simulink model "Main1"  (R2017b)
settings: Solver=ode15s  StartTime=0.0  StopTime=t_end  FixedStep=.0001  MaxStep=st  RelTol=1e-3  EnableMultiTasking=on
values from neighbouring files (symbols this model uses):
  A = eye(16,16)    [full_input_list.m]
  B = zeros(16,1)    [full_input_list.m]
  C = blkdiag(eye(3,3),zeros(3,3),eye(10,10))    [full_input_list.m]
  deltaT = 0.00001    (= 1e-05)    [full_input_list.m]
  H = C    [full_input_list.m]
  I_UD = [0.032808359, 0.000617048, 0.000049185;      0.000617048, 0.032531573, 0.000060042;      0.000049185, 0.000060042, 0.007799591]    [full_input_list.m]
  kd = 0.5    [full_input_list.m]    (also in initACS.m = 0.01)
  kd_UD_detumble = 6e-3    (= 0.006)    [full_input_list.m]
  kd_UD_slew = epsilon_UD_slew*.3    (= 0.003)    [full_input_list.m]
  kd_UD_spinUp = epsilon_UD_spinUp*0.025    (= 0.00025)    [full_input_list.m]
  kp = 1    [full_input_list.m]    (also in initACS.m = 0.01)
  kp_UD_slew = epsilon_UD_slew^2*.01    (= 1e-06)    [full_input_list.m]
  kp_UD_spinUp = epsilon_UD_spinUp^2*.05    (= 5e-06)    [full_input_list.m]
  magMomentMax_B = sat2CoilArea.*sat2n.*currentMax_B    [full_input_list.m]
  omega_cmd_N = 1e-1*[1 1 -.6]'    [full_input_list.m]
  omega_spinUp_MAG = 0.05    [full_input_list.m]
  OpModes = [0 0 0]    [full_input_list.m]
  OpTimes = [0 1 2]    [full_input_list.m]
  q4_cmd_init = [q4_cmd_init(2:4); q4_cmd_init(1)]    [full_input_list.m]
  Q_k = zeros(16,16)    [full_input_list.m]
  R = R_k    [full_input_list.m]
  sat2CoilArea = 0.8*[0.02; 0.02; 0.01]    [full_input_list.m]
  sat2n = [0; 100; 100]    [full_input_list.m]
  sat2Resistance = sat2WireLength.*sat2WireResistivity./sat2WireArea    [full_input_list.m]
  SeperationTime = 30000    [full_input_list.m]
  spinAxis_B = [1 0 0]    [full_input_list.m]
  st = 1/freq    (= 0.0125)    [full_input_list.m]    (also in initSimulink.m)
  u_k = zeros(16,1)    [full_input_list.m]
  w_k = zeros(16,1)    [full_input_list.m]
  Z_k = zeros(16,1)    [full_input_list.m]
undefined symbols (not defined in the file or in its folder): DiscIntNeverNeededParam, G_igrf, gyro_DCM_BS, H_igrf, I_B, IAU, Kschmidt, mag_variance, R_mean
libraries: aerolibutil x36, vrlib x31, SimMainLibrary x27, simulink x22, dspmathops x6, sharedtransform x4, sharedutil x2, dspinverses x2, dspmtrx3 x1, aerolibtransform2 x1, aerolibgravity2 x1, lib_violet_env x1
(part 1 of 3)
settings Model: Creator=dtk42  LastModifiedBy=vtroo
settings SolverCC: ZeroCrossAlgorithm=Adaptive
settings OptimizationCC: LifeSpan=inf
settings DebuggingCC: SFUnexpectedBacktrackingDiag=warning  SFNoUnconditionalDefaultTransitionDiag=warning  SFExecutionAtInitializationDiag=none
settings CodeAppCC: StateflowObjectComments=on
settings GRTTargetCC: TargetLangStandard=C89/C90 (ANSI)
settings ConfigComp: CovMetricSettings=dw  CovHtmlReporting=on  CovSaveCumulativeToWorkspaceVar=on  CovSaveSingleToWorkspaceVar=on  CovExternalEMLEnable=off
settings SimscapeCC: SimscapeNormalizeSystem=off
settings ExplorerConfigSet: InternalSimMechanicsExplorerSettings="<ExplorerConfiguration><canonicalview>default</canonicalview><AnimationSetting><BasePlaybackSpeed>1.0</BasePlaybackSpeed><PlaybackSpeedFactor>0.125</PlaybackSpeedFactor></AnimationSetting><TilePanel><TileInfo><Tiles Columns=\"1\" Count=\"1\" Rows=\"1\"><Column Weight=\"1\"/><Row Weight=\"1\"/><Tile Height=\"1\" Width=\"1\" X=\"0\" Y=\"0\"/></Tiles></TileInfo><SceneInfo><SceneViewer><BGColor><R>0.60000002384185791</R><G>0.60000002384185791</G><B>0.60000002384185791</B></BGColor><Camera><DoPerspective>on</DoPerspective><Position><X>0.299996941150711738</X><Y>-0.0249603631658691372</Y><Z>0.248754528744442288</Z></Position><Center><X>-0.199992462724818743</X><Y>0.0615041817400976409</Y><Z>-0.612949874450989807</Z></Center><Up><X>0.866031521373320734</X><Y>0.049918851895640326</Y><Z>-0.49749121822724951</Z></Up><ViewLimDist>1</ViewLimDist><YLim>0.466307658154998583</YLim><XLim>1.03172600323492714</XLim></Camera></SceneViewer></SceneInfo></TilePanel><MechEditorPanel><Cameras><Camera><Id>Camera1</Id><Value><Name>Camera1</Name><NativeCamera><PositionTrackingFeature>Dynamics_Configurable_System1.Three_Link_Simscape_Model.Camera1_Frame.F</PositionTrackingFeature><CenterTrackingFeature>Dynamics_Configurable_System1.Three_Link_Simscape_Model.Camera1_Frame.F</CenterTrackingFeature><UpVectorTrackingFeature>Dynamics_Configurable_System1.Three_Link_Simscape_Model.Camera1_Frame.F</UpVectorTrackingFeature><CenterTrackingOrigin>off</CenterTrackingOrigin><CenterTrackingDirection>-Z</CenterTrackingDirection><UpVectorTrackingDirection>+X</UpVectorTrackingDirection></NativeCamera></Value></Camera></Cameras><GfxPanelCameraMap><MapElement CameraMLId=\"Camera1\" GfxPanelIndex=\"0\"/></GfxPanelCameraMap><VideoCreator><PlaybackSpeedRatio>0.25</PlaybackSpeedRatio><FrameRate>30</FrameRate><VideoFormat>Motion JPEG AVI</VideoFormat><FrameSize>[800 600]</FrameSize></VideoCreator></MechEditorPanel></ExplorerConfiguration>"

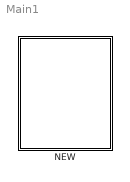
== system Main1 ==
  NEW : Subsystem

== system Main1/NEW ==
  note: CUGravity Top Level Simulation
  note: Feeding exact telemetry from dynamics into FC. Substitute this for EKF output until estimation is ready for implementation.
  Dynamics Configurable System2 : Subsystem  BlockChoice=Three Link Simscape Model
      link override Extendable Single  Link Simscape /s_teth_init2: PxPositionTargetSpecify=on  PxPositionTargetValue=eps
      link override Single Link Simscape Model/s_teth_init: PxPositionTargetSpecify=on  PxPositionTargetValue=eps  PyPositionTargetSpecify=on  PyPositionTargetValue=eps  PzPositionTargetSpecify=on  PzPositionTargetValue=eps
      link override Single Link Simscape Model/s_teth_init2: PxPositionTargetSpecify=on  PxPositionTargetValue=eps  PyPositionTargetSpecify=on  PyPositionTargetValue=eps  PzPositionTargetSpecify=on  PzPositionTargetValue=eps
      link override Three Link Simscape Model/Kane Damper 1: SerializedFrames=<Frames><Frame><Id>Frame1</Id><Value><Name>F1</Name><Origin><Source>GeometricFeature</Source><FeatureName>+z surface</FeatureName></Origin><PrimaryAxis><DefinedDirection>+Z</DefinedDirection><Source>ReferenceFrame</Source><SourceDirection>+Z</SourceDirection><FeatureName></FeatureName></PrimaryAxis><SecondaryAxis><DefinedDirection>+X</DefinedDirection><Source>ReferenceFrame</Source><SourceDirection>+X</SourceDirection><FeatureName></FeatureName></SecondaryAxis></Value></Frame></Frames>
      link override Three Link Simscape Model/Kane Damper 2: SerializedFrames=<Frames><Frame><Id>Frame1</Id><Value><Name>F1</Name><Origin><Source>GeometricFeature</Source><FeatureName>-z surface</FeatureName></Origin><PrimaryAxis><DefinedDirection>+Z</DefinedDirection><Source>ReferenceFrame</Source><SourceDirection>+Z</SourceDirection><FeatureName></FeatureName></PrimaryAxis><SecondaryAxis><DefinedDirection>+X</DefinedDirection><Source>ReferenceFrame</Source><SourceDirection>+X</SourceDirection><FeatureName></FeatureName></SecondaryAxis></Value></Frame></Frames>  GeometryShape=Brick  BrickDimensions=[kane_radius kane_radius kane_height]
      link override Undeployed Model/Center Sat1: GraphicDiffuseColor=[0.0 0.8 0.8]  GraphicOpacity=.5  SerializedFrames=<Frames><Frame><Id>Frame1</Id><Value><Name>PosZ</Name><Origin><Source>GeometricFeature</Source><FeatureName>+z surface</FeatureName></Origin><PrimaryAxis><DefinedDirection>+Z</DefinedDirection><Source>ReferenceFrame</Source><SourceDirection>+Z</SourceDirection><FeatureName></FeatureName></PrimaryAxis><SecondaryAxis><DefinedDirection>+X</DefinedDirection><Source>ReferenceFrame</Source><SourceDirection>+X</SourceDirection><FeatureName></FeatureName></SecondaryAxis></Value></Frame><Frame><Id>Frame2</Id><Value><Name>NegZ</Name><Origin><Source>GeometricFeature</Source><FeatureName>-z surface</FeatureName></Origin><PrimaryAxis><DefinedDirection>+Z</DefinedDirection><Source>ReferenceFrame</Source><SourceDirection>+Z</SourceDirection><FeatureName></FeatureName></PrimaryAxis><SecondaryAxis><DefinedDirection>+X</DefinedDirection><Source>ReferenceFrame</Source><SourceDirection>+X</SourceDirection><FeatureName></FeatureName></SecondaryAxis></Value></Frame><Frame><Id>Frame7</Id><Value><Name>PosX</Name><Origin><Source>GeometricFeature</Source><FeatureName>+x surface</FeatureName></Origin><PrimaryAxis><DefinedDirection>+Z</DefinedDirection><Source>ReferenceFrame</Source><SourceDirection>+Z</SourceDirection><FeatureName></FeatureName></PrimaryAxis><SecondaryAxis><DefinedDirection>+X</DefinedDirection><Source>ReferenceFrame</Source><SourceDirection>+X</SourceDirection><FeatureName></FeatureName></SecondaryAxis></Value></Frame><Frame><Id>Frame8</Id><Value><Name>COM</Name><Origin><Source>CenterOfMassFrame</Source><FeatureName></FeatureName></Origin><PrimaryAxis><DefinedDirection>+Z</DefinedDirection><Source>ReferenceFrame</Source><SourceDirection>+Z</SourceDirection><FeatureName></FeatureName></PrimaryAxis><SecondaryAxis><DefinedDirection>+X</DefinedDirection><Source>ReferenceFrame</Source><SourceDirection>+X</SourceDirection><FeatureName></FeatureName></SecondaryAxis></Value></Frame></Frames>
      link override Undeployed Model/EndSat3: GraphicOpacity=.5  GraphicDiffuseColor=[1.0 0.0 0.0]
      link override Undeployed Model/EndSat4: GraphicOpacity=.5  GraphicDiffuseColor=[1.0 0.0 0.0]
      settings: AttributesFormatString=%<BlockChoice>  TemplateBlock=SimMainLibrary/Dynamics Configurable System  MemberBlocks="Extendable Single  Link Simscape ,Single Link Simscape Model,Three Link Simscape Model,Undeployed Model"
  Flight Computers1 : Subsystem
  Memory2 : Memory  InheritSampleTime=on
  Memory3 : Memory  InheritSampleTime=on
  Rate Transition3 : RateTransition  OutPortSampleTime=st
  Rate Transition4 : RateTransition  OutPortSampleTime=st
  Scope : Scope
  Scopes1 : Subsystem
  Sensors1 : Subsystem  mask(State Estimation){}
      mask help: This block uses the plant model calculated state (input) and adds sensor noise to the system to calculate the estimated state (output). The middle satellite has a more extensive set of calculations required to complete the state estimation, than do the end satellites. All three satellites compute the accelerometer, magnetometer, angular velocity, and sun sensor vector measurements. The middle satellite performs additional calculations to accurately measure simulation time and inertial position of the center of mass.
  To Workspace3 : ToWorkspace  VariableName=stateArr1  SaveFormat=Timeseries  SampleTime=-1
  To Workspace5 : ToWorkspace  VariableName=stateEstimation1  SaveFormat=Timeseries  SampleTime=-1
  wires:
  Dynamics Configurable System2/1(State k+1) -> To Workspace3/1, Memory2/1, Scopes1/2(state)
  Flight Computers1/2(PwbMEX) -> Memory3/1
  Dynamics Configurable System2/2(DEBUG) -> Scope/1
  Rate Transition4/1 -> Flight Computers1/2(TEMP_State)
  Flight Computers1/3(StateEst) -> To Workspace5/1
  Rate Transition3/1 -> Flight Computers1/1(Sensor Data)
  Sensors1/1(Observation) -> Rate Transition3/1
  Memory2/1 -> Sensors1/1(State), Rate Transition4/1
  Flight Computers1/1(FC Outputs) -> Dynamics Configurable System2/1(Actuation Cmds), Scopes1/1(torque_N)
  Memory3/1 -> Flight Computers1/3(PwbMEXin)

== system Main1/NEW/Dynamics Configurable System2 ==
  Actuation Cmds : Inport
  Three Link Simscape Model : SimMainLibrary/Three Link Simscape Model
      settings: SourceProductName=CUGravity Library
  State k+1 : Outport
  DEBUG : Outport  Port=2
  wires:
  Actuation Cmds/1 -> Three Link Simscape Model/1
  Three Link Simscape Model/1 -> State k+1/1
  Three Link Simscape Model/2 -> DEBUG/1

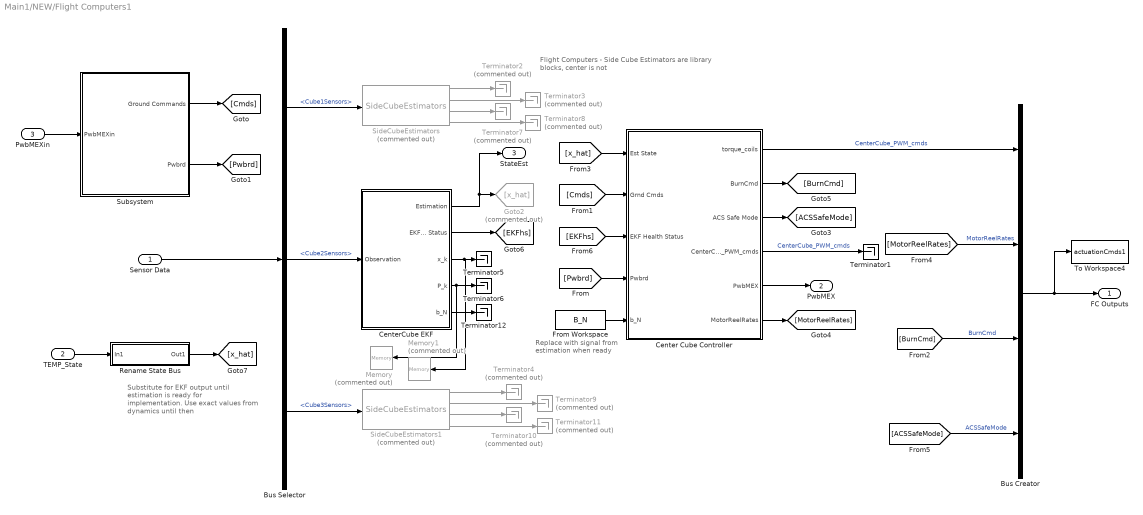
== system Main1/NEW/Flight Computers1 ==
  note: Substitute for EKF output until estimation is ready for implementation. Use exact values from dynamics until then
  note: Flight Computers
      | - Side Cube Estimators are library blocks, center is not
  note: Replace with signal from estimation when ready
  Sensor Data : Inport
  TEMP_State : Inport  Port=2
  PwbMEXin : Inport  Port=3
  Bus Creator : BusCreator  Inputs=4
  Bus Selector : BusSelector  OutputSignals=Cube1Sensors,Cube2Sensors,Cube3Sensors
  Center Cube Controller : Subsystem
  CenterCube EKF : Subsystem
  From Workspace : FromWorkspace  VariableName=B_N  SampleTime=0
  Goto2 : Goto  Commented=on  GotoTag=x_hat
  Memory : Memory  Commented=on
  Memory1 : Memory  Commented=on
  Rename State Bus : Subsystem
  SideCubeEstimators : SimMainLibrary/SideCubeEstimators  Commented=on
      settings: SourceProductName=CUGravity Library
  SideCubeEstimators1 : SimMainLibrary/SideCubeEstimators  Commented=on
      settings: SourceProductName=CUGravity Library
  Subsystem : Subsystem
  Terminator{1,5..6,12} (4 alike) : Terminator
  Terminator{2..4,7..11} (8 alike) : Terminator  Commented=on
  To Workspace4 : ToWorkspace  VariableName=actuationCmds1  SaveFormat=Timeseries  SampleTime=-1
  FC Outputs : Outport
  PwbMEX : Outport  Port=2
  StateEst : Outport  Port=3
  wires:
  Sensor Data/1 -> Bus Selector/1
  Bus Selector/1 -> SideCubeEstimators/1  "<Cube1Sensors>"
  Bus Selector/2 -> CenterCube EKF/1(Observation)  "<Cube2Sensors>"
  Bus Selector/3 -> SideCubeEstimators1/1  "<Cube3Sensors>"
  SideCubeEstimators/1 -> Terminator2/1
  Bus Creator/1 -> To Workspace4/1, FC Outputs/1
  Subsystem/1(Ground Commands) -> [Cmds]
  [Cmds] -> Center Cube Controller/2(Grnd Cmds)
  Center Cube Controller/3(ACS Safe Mode) -> [ACSSafeMode]
  Center Cube Controller/2(BurnCmd) -> [BurnCmd]
  [BurnCmd] -> Bus Creator/3  "BurnCmd"
  CenterCube EKF/2(EKF Health Status) -> [EKFhs]
  [EKFhs] -> Center Cube Controller/3("EKF Health Status ")
  Subsystem/2(Pwbrd) -> [Pwbrd]
  [Pwbrd] -> Center Cube Controller/4(Pwbrd)
  Center Cube Controller/5(PwbMEX) -> PwbMEX/1
  CenterCube EKF/1(Estimation) -> Goto2/1, StateEst/1
  [x_hat] -> Center Cube Controller/1(Est State)
  Center Cube Controller/4(CenterCube_PWM_cmds) -> Terminator1/1  "CenterCube_PWM_cmds"
  SideCubeEstimators/2 -> Terminator3/1
  CenterCube EKF/3(x_k) -> Memory1/1, Terminator5/1
  CenterCube EKF/4(P_k) -> Terminator6/1, Memory/1
  SideCubeEstimators/3 -> Terminator7/1
  SideCubeEstimators/4 -> Terminator8/1
  SideCubeEstimators1/1 -> Terminator4/1
  SideCubeEstimators1/2 -> Terminator9/1
  SideCubeEstimators1/3 -> Terminator10/1
  SideCubeEstimators1/4 -> Terminator11/1
  [ACSSafeMode] -> Bus Creator/4  "ACSSafeMode"
  Center Cube Controller/6(MotorReelRates) -> [MotorReelRates]
  [MotorReelRates] -> Bus Creator/2  "MotorReelRates"
  Center Cube Controller/1(torque_coils) -> Bus Creator/1  "CenterCube_PWM_cmds"
  From Workspace/1 -> Center Cube Controller/5(b_N)
  CenterCube EKF/5(b_N) -> Terminator12/1
  TEMP_State/1 -> Rename State Bus/1(In1)
  Rename State Bus/1(Out1) -> [x_hat]
  PwbMEXin/1 -> Subsystem/1(PwbMEXin)

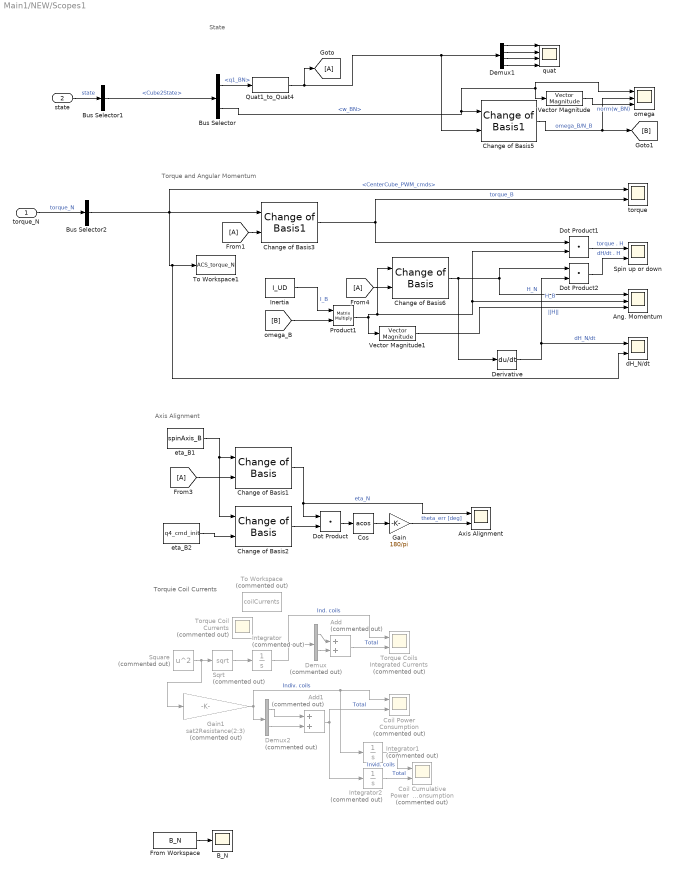
== system Main1/NEW/Scopes1 ==
  note: State
  note: Torque and Angular Momentum
  note: Axis Alignment
  note: Torquie Coil Currents
  torque_N : Inport
  state : Inport  Port=2
  Add : Sum  Commented=on
  Add1 : Sum  Commented=on
  Ang. Momentum : Scope  NumInputPorts=3
  Axis Alignment : Scope  NumInputPorts=2
  B_N : Scope
  Bus Selector : BusSelector  OutputSignals=q1_BN,w_BN
  Bus Selector1 : BusSelector  OutputSignals=Cube2State
  Bus Selector2 : BusSelector  OutputSignals=CenterCube_PWM_cmds
  Change of Basis1 : SimMainLibrary/Change of Basis
      settings: SourceProductName=CUGravity Library
  Change of Basis2 : SimMainLibrary/Change of Basis
      settings: SourceProductName=CUGravity Library
  Change of Basis3 : SimMainLibrary/Change of Basis1
      settings: SourceProductName=CUGravity Library
  Change of Basis5 : SimMainLibrary/Change of Basis1
      settings: SourceProductName=CUGravity Library
  Change of Basis6 : SimMainLibrary/Change of Basis
      settings: SourceProductName=CUGravity Library
  Coil Cumulative Power  Consumption : Scope  Commented=on  NumInputPorts=2
  Coil Power Consumption : Scope  Commented=on  NumInputPorts=2
  Cos : Trigonometry  Operator=acos
  Demux : Demux  Commented=on  Outputs=2
  Demux1 : Demux
  Demux2 : Demux  Commented=on  Outputs=2
  Derivative : Derivative
  Dot Product : DotProduct  InputSameDT=on  OutDataTypeStr=Inherit: Inherit via internal rule
  Dot Product1 : DotProduct  InputSameDT=on  OutDataTypeStr=Inherit: Inherit via internal rule
  Dot Product2 : DotProduct  InputSameDT=on  OutDataTypeStr=Inherit: Inherit via internal rule
  From Workspace : FromWorkspace  VariableName=B_N  SampleTime=0
  Gain : Gain  Gain=180/pi
  Gain1 : Gain  Commented=on  Gain=sat2Resistance(2:3)
  Inertia : Constant  Value=I_UD
  Integrator : Integrator  Commented=on
  Integrator1 : Integrator  Commented=on
  Integrator2 : Integrator  Commented=on
  Product1 : Product  Multiplication=Matrix(*)
  Quat1_to_Quat4 : SimMainLibrary/Quat1_to_Quat4
      settings: SourceProductName=CUGravity Library
  Spin up or down : Scope  NumInputPorts=2
  Sqrt : Sqrt  Commented=on  SaturateOnIntegerOverflow=on
  Square : Math  Commented=on  Operator=square  RndMeth=Zero  SaturateOnIntegerOverflow=on
  To Workspace : ToWorkspace  Commented=on  VariableName=coilCurrents  SaveFormat=Timeseries  SampleTime=-1
  To Workspace1 : ToWorkspace  VariableName=ACS_torque_N  SaveFormat=Timeseries  SampleTime=-1
  Torque Coil Currents : Scope  Commented=on
  Torque Coils Integrated Currents : Scope  Commented=on  NumInputPorts=2
  Vector Magnitude : SimMainLibrary/Vector Magnitude
      settings: SourceProductName=CUGravity Library
  Vector Magnitude1 : SimMainLibrary/Vector Magnitude
      settings: SourceProductName=CUGravity Library
  dH_N/dt : Scope  NumInputPorts=2
  eta_B1 : Constant  Value=spinAxis_B
  eta_B2 : Constant  Value=q4_cmd_init
  omega : Scope  NumInputPorts=3
  quat : Scope  NumInputPorts=4
  torque : Scope  NumInputPorts=2
  wires:
  ? -> To Workspace/1, Square/1, Torque Coil Currents/1
  Integrator/1 -> Demux/1, Torque Coils Integrated Currents/1  "Ind. coils"
  Cos/1 -> Gain/1
  Change of Basis1/1 -> Dot Product/1, Axis Alignment/1  "eta_N"
  eta_B1/1 -> Change of Basis2/1, Change of Basis1/1
  Change of Basis2/1 -> Dot Product/2
  eta_B2/1 -> Change of Basis2/2
  [A] -> Change of Basis1/2
  Dot Product/1 -> Cos/1
  Gain/1 -> Axis Alignment/2  "theta_err [deg]"
  Bus Selector2/1 -> dH_N/dt/2, To Workspace1/1, torque/1, Change of Basis3/1  "<CenterCube_PWM_cmds>"
  [B] -> Product1/2
  Dot Product1/1 -> Spin up or down/1  "torque . H"
  Derivative/1 -> dH_N/dt/1, Dot Product2/2  "dH_N/dt"
  Vector Magnitude1/1 -> Ang. Momentum/3  "||H||"
  [A] -> Change of Basis3/2
  Product1/1 -> Change of Basis6/1, Ang. Momentum/2, Dot Product1/2, Vector Magnitude1/1  "H_B"
  Inertia/1 -> Product1/1  "I_B"
  Change of Basis3/1 -> Dot Product1/1, torque/2  "torque_B"
  [A] -> Change of Basis6/2
  Change of Basis6/1 -> Derivative/1, Dot Product2/1, Ang. Momentum/1  "H_N"
  Demux1/2 -> quat/2
  Demux1/3 -> quat/3
  Demux1/4 -> quat/4
  Bus Selector/2 -> Change of Basis5/1, Vector Magnitude/1, omega/1  "<w_BN>"
  Change of Basis5/1 -> omega/2, [B]  "omega_B/N_B"
  Bus Selector/1 -> Quat1_to_Quat4/1  "<q1_BN>"
  Vector Magnitude/1 -> omega/3  "norm(w_BN)"
  Demux1/1 -> quat/1
  Square/1 -> Gain1/1, Sqrt/1
  Sqrt/1 -> Integrator/1
  Demux/1 -> Add/1
  Demux/2 -> Add/2
  Add/1 -> Torque Coils Integrated Currents/2  "Total"
  Gain1/1 -> Integrator1/1, Coil Power Consumption/1, Demux2/1  "Indiv. coils"
  Demux2/1 -> Add1/1
  Demux2/2 -> Add1/2
  Add1/1 -> Integrator2/1, Coil Power Consumption/2  "Total"
  Integrator1/1 -> Coil Cumulative Power  Consumption/1  "Invid. coils"
  Integrator2/1 -> Coil Cumulative Power  Consumption/2  "Total"
  state/1 -> Bus Selector1/1  "state"
  Bus Selector1/1 -> Bus Selector/1  "<Cube2State>"
  Quat1_to_Quat4/1 -> [A], Change of Basis5/2, Demux1/1
  torque_N/1 -> Bus Selector2/1  "torque_N"
  Dot Product2/1 -> Spin up or down/2  "dH/dt . H"
  From Workspace/1 -> B_N/1

== system Main1/NEW/Sensors1 ==
  State : Inport
  Bus Creator1 : BusCreator  Inputs=3
  Bus Selector1 : BusSelector  OutputSignals=Cube1State,Cube2State,Cube3State
  Center Cube Sensors : Subsystem
  EndSat Sensor1 : Subsystem
  EndSat Sensor2 : Subsystem
  Observation : Outport
  wires:
  Bus Creator1/1 -> Observation/1
  Bus Selector1/1 -> EndSat Sensor2/1(State)  "<Cube1State>"
  EndSat Sensor2/1(Sensors) -> Bus Creator1/1  "Cube1Sensors"
  EndSat Sensor1/1(Sensors) -> Bus Creator1/3  "Cube3Sensors"
  Center Cube Sensors/1(Sensors) -> Bus Creator1/2  "Cube2Sensors"
  Bus Selector1/2 -> Center Cube Sensors/1(State)  "<Cube2State>"
  Bus Selector1/3 -> EndSat Sensor1/1(State)  "<Cube3State>"
  State/1 -> Bus Selector1/1

== system Main1/NEW/Flight Computers1/Center Cube Controller ==
  note: Why does torque coils suddenly become PWM?
  Est State : Inport
  Grnd Cmds : Inport  Port=2
  "EKF Health Status " : Inport  Port=3
  Pwbrd : Inport  Port=4
  b_N : Inport  Port=5
  Attitude Compensator : Subsystem
  Bus Selector : BusSelector  OutputSignals=w_BN_est
  Memory : Memory  InheritSampleTime=on
  Motor Control Placeholder : Subsystem  Commented=on
  Motor Controller Scope : Scope
  SafeMode : Subsystem
  "Sequential Motor Controller " : SimMainLibrary/Sequential Motor Controller
      settings: SourceProductName=CUGravity Library
  Terminator1 : Terminator
  Terminator2 : Terminator
  Terminator3 : Terminator
  Torque Coil Management : Subsystem
  torque_coils : Outport
  BurnCmd : Outport  Port=2
  ACS Safe Mode : Outport  Port=3
  CenterCube_PWM_cmds : Outport  Port=4
  PwbMEX : Outport  Port=5
  MotorReelRates : Outport  Port=6
  wires:
  Memory/1 -> SafeMode/3(Safe Mode In)
  Attitude Compensator/2(SepBurn) -> BurnCmd/1
  SafeMode/2(SafedSeperationBurn) -> Attitude Compensator/2(SafedSepBurn)
  SafeMode/3(SafedPos) -> Terminator3/1
  SafeMode/4(SafedVel) -> Terminator2/1
  Est State/1 -> SafeMode/2(EstState)
  SafeMode/1(SafedOpMode) -> "Sequential Motor Controller "/2, Motor Control Placeholder/2(SafedOpMode), Attitude Compensator/1(SafedOpMode)
  Grnd Cmds/1 -> SafeMode/1(GrndCmds)
  "EKF Health Status "/1 -> SafeMode/5("EKFhs ")
  Pwbrd/1 -> SafeMode/4(Pwbrd)
  Torque Coil Management/2(torque_coils) -> torque_coils/1
  Torque Coil Management/1(CenterCube_PWM_cmds) -> CenterCube_PWM_cmds/1
  Attitude Compensator/3(torque_N) -> Torque Coil Management/2(torque_N)
  SafeMode/5(Safed Att. State) -> Bus Selector/1, Torque Coil Management/1(Att. State), Attitude Compensator/3(Att. State)
  SafeMode/6(Safe Mode Out) -> Memory/1, ACS Safe Mode/1
  SafeMode/7(PwbMEX) -> PwbMEX/1
  Attitude Compensator/1(OpMode) -> Terminator1/1
  "Sequential Motor Controller "/1 -> MotorReelRates/1
  "Sequential Motor Controller "/2 -> Motor Controller Scope/1
  b_N/1 -> [B_N]
  [B_N] -> Attitude Compensator/4(B_N)
  [B_N] -> Torque Coil Management/3(B_N)
  Bus Selector/1 -> "Sequential Motor Controller "/1  "<w_BN_est>"

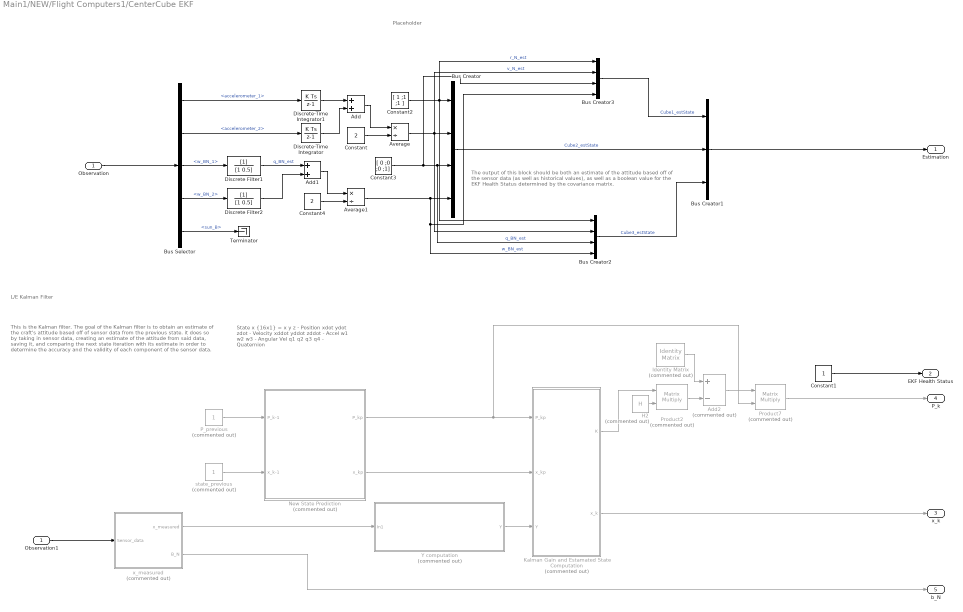
== system Main1/NEW/Flight Computers1/CenterCube EKF ==
  note: The output of this block should be both an estimate of the attitude based off of the sensor data (as well as historical values), as well as a boolean value for the EKF Health Status determined by the covariance matrix.
  note: Placeholder
  note: This is the Kalman filter. The goal of the Kalman filter is to obtain an estimate of the craft's attitude based off of sensor data from the previous state. it does so by taking in sensor data, creating an estimate of the attitude from said data, saving it, and comparing the next state iteration with its estimate in order to determine the accuracy and the validity of each component of the sensor data.
  note: L/E Kalman Filter
  note: State x {16x1} =
      | x y z - Position
      | xdot ydot zdot - Velocity
      | xddot yddot zddot - Accel
      | w1 w2 w3 - Angular Vel
      | q1 q2 q3 q4 - Quaternion
  Observation : Inport
  Add : Sum
  Add1 : Sum
  Add2 : Sum  Commented=on  Inputs=+-
  Average : Product  Inputs=*/
  Average1 : Product  Inputs=*/
  Bus Creator : BusCreator  Inputs=4
  Bus Creator1 : BusCreator  Inputs=3
  Bus Creator2 : BusCreator  Inputs=4
  Bus Creator3 : BusCreator  Inputs=4
  Bus Selector : BusSelector  OutputSignals=accelerometer_1,accelerometer_2,w_BN_1,w_BN_2,sun_B
  Constant : Constant  Value=2
  Constant1 : Constant
  Constant2 : Constant  Value=[ 1 ;1 ;1 ]
  Constant3 : Constant  Value=[ 0 ;0 ;0 ;1]
  Constant4 : Constant  Value=2
  Discrete Filter1 : DiscreteFilter
  Discrete Filter2 : DiscreteFilter
  Discrete-Time Integrator : DiscreteIntegrator  InitialConditionSetting=State (most efficient)  SampleTime=-1  ICPrevOutput=DiscIntNeverNeededParam  ICPrevScaledInput=DiscIntNeverNeededParam
  Discrete-Time Integrator1 : DiscreteIntegrator  InitialConditionSetting=State (most efficient)  SampleTime=-1  ICPrevOutput=DiscIntNeverNeededParam  ICPrevScaledInput=DiscIntNeverNeededParam
  H2 : Constant  Commented=on  Value=H
  Identity Matrix : dspmtrx3/Identity Matrix  Commented=on  Inherit=off  N=16  Ts=1  dataType=double  isSigned=on  wordLen=16  udDataType=sfix(16)  fracBitsMode=Best precision  numFracBits=15  OutDataTypeStr=double  LastOutDataTypeStr=double
      settings: SourceProductName=DSP System Toolbox
  Kalman Gain and Estamated State Computation : Subsystem  Commented=on
  "New State Prediction " : Subsystem  Commented=on
  Observation1 : InportShadow
  P_previous : Constant  Commented=on
  Product2 : Product  Commented=on  Multiplication=Matrix(*)
  Product7 : Product  Commented=on  Multiplication=Matrix(*)
  Terminator : Terminator
  Y computation : Subsystem  Commented=on
  state_previous : Constant  Commented=on
  x_measured : Subsystem  Commented=on
  Estimation : Outport
  EKF Health Status : Outport  Port=2
  x_k : Outport  Port=3
  P_k : Outport  Port=4
  b_N : Outport  Port=5
  wires:
  Bus Selector/2 -> Discrete-Time Integrator/1  "<accelerometer_2>"
  Discrete-Time Integrator/1 -> Add/2
  Bus Selector/4 -> Discrete Filter2/1  "<w_BN_2>"
  Add/1 -> Average/1
  Constant/1 -> Average/2
  Average/1 -> Bus Creator3/2, Bus Creator2/2, Bus Creator/2  "v_N_est"
  Bus Selector/1 -> Discrete-Time Integrator1/1  "<accelerometer_1>"
  Bus Selector/3 -> Discrete Filter1/1  "<w_BN_1>"
  Observation/1 -> Bus Selector/1
  Bus Creator/1 -> Bus Creator1/2  "Cube2_estState"
  Constant3/1 -> Bus Creator3/3, Bus Creator2/3, Bus Creator/3  "q_BN_est"
  Constant2/1 -> Bus Creator3/1, Bus Creator2/1, Bus Creator/1  "r_N_est"
  Average1/1 -> Bus Creator2/4, Bus Creator3/4, Bus Creator/4  "w_BN_est"
  Bus Selector/5 -> Terminator/1  "<sun_B>"
  Discrete-Time Integrator1/1 -> Add/1
  Discrete Filter2/1 -> Add1/2
  Add1/1 -> Average1/1
  Constant4/1 -> Average1/2
  Discrete Filter1/1 -> Add1/1  "q_BN_est"
  Bus Creator1/1 -> Estimation/1
  Bus Creator3/1 -> Bus Creator1/1  "Cube1_estState"
  Bus Creator2/1 -> Bus Creator1/3  "Cube3_estState"
  Constant1/1 -> EKF Health Status/1
  P_previous/1 -> "New State Prediction "/1(P_k-1)
  state_previous/1 -> "New State Prediction "/2(x_k-1)
  "New State Prediction "/1(P_kp) -> Product7/2, Kalman Gain and Estamated State Computation/1(P_kp)
  Kalman Gain and Estamated State Computation/2(x_k) -> x_k/1
  Identity Matrix/1 -> Add2/1
  H2/1 -> Product2/2
  Product2/1 -> Add2/2
  Add2/1 -> Product7/1
  Product7/1 -> P_k/1
  Kalman Gain and Estamated State Computation/1(K) -> Product2/1
  "New State Prediction "/2("x_kp  ") -> Kalman Gain and Estamated State Computation/2(x_kp)
  Y computation/1(Y) -> Kalman Gain and Estamated State Computation/3(Y)
  x_measured/1(x_measured) -> Y computation/1(In1)
  x_measured/2(B_N) -> b_N/1
  Observation1/1 -> x_measured/1(Sensor_data)

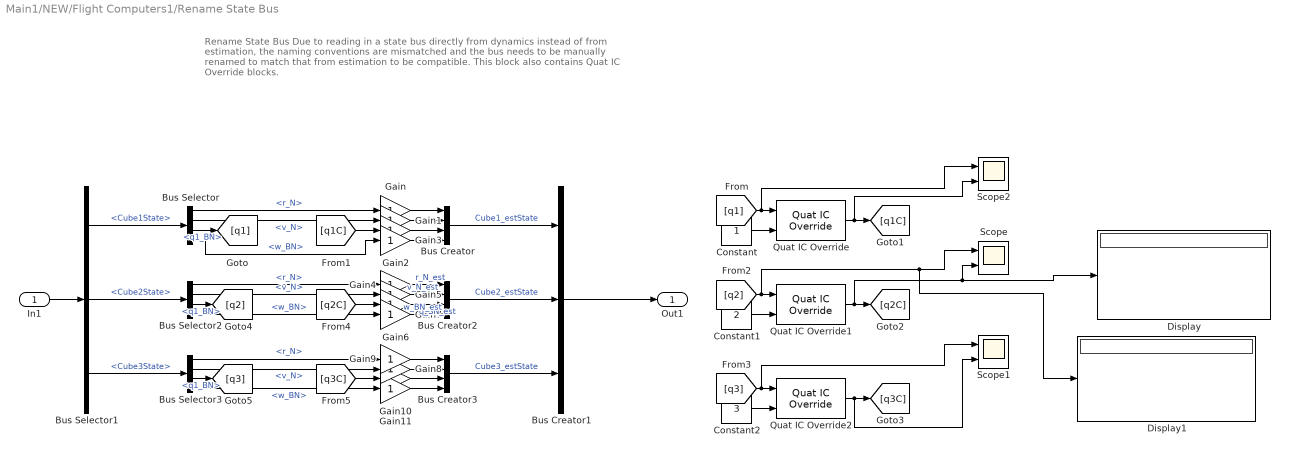
== system Main1/NEW/Flight Computers1/Rename State Bus ==
  note: Rename State Bus
      | Due to reading in a state bus directly from dynamics instead of from estimation, the naming conventions are mismatched and the bus needs to be manually renamed to match that from estimation to be compatible.
      | This block also contains Quat IC Override blocks.
  In1 : Inport
  Bus Creator : BusCreator  Inputs=4
  Bus Creator1 : BusCreator  Inputs=3
  Bus Creator2 : BusCreator  Inputs=4
  Bus Creator3 : BusCreator  Inputs=4
  Bus Selector : BusSelector  OutputSignals=r_N,v_N,q1_BN,w_BN
  Bus Selector1 : BusSelector  OutputSignals=Cube1State,Cube2State,Cube3State
  Bus Selector2 : BusSelector  OutputSignals=r_N,v_N,q1_BN,w_BN
  Bus Selector3 : BusSelector  OutputSignals=r_N,v_N,q1_BN,w_BN
  Constant : Constant
  Constant1 : Constant  Value=2
  Constant2 : Constant  Value=3
  Display : Display
  Display1 : Display
  Gain{,1..11} (12 alike) : Gain
  Quat IC Override : SimMainLibrary/Quat IC Override
      settings: SourceProductName=CUGravity Library
  Quat IC Override1 : SimMainLibrary/Quat IC Override
      settings: SourceProductName=CUGravity Library
  Quat IC Override2 : SimMainLibrary/Quat IC Override
      settings: SourceProductName=CUGravity Library
  Scope : Scope  NumInputPorts=2
  Scope1 : Scope  NumInputPorts=2
  Scope2 : Scope  NumInputPorts=2
  Out1 : Outport
  wires:
  In1/1 -> Bus Selector1/1
  Bus Selector1/2 -> Bus Selector2/1  "<Cube2State>"
  Bus Selector1/1 -> Bus Selector/1  "<Cube1State>"
  Bus Creator1/1 -> Out1/1
  Bus Selector1/3 -> Bus Selector3/1  "<Cube3State>"
  Bus Selector/1 -> Gain/1  "<r_N>"
  Bus Selector/2 -> Gain1/1  "<v_N>"
  Bus Creator/1 -> Bus Creator1/1  "Cube1_estState"
  Bus Selector2/4 -> Gain7/1  "<w_BN>"
  Bus Selector2/2 -> Gain5/1  "<v_N>"
  Bus Selector2/1 -> Gain4/1  "<r_N>"
  Bus Creator2/1 -> Bus Creator1/2  "Cube2_estState"
  Bus Selector3/1 -> Gain9/1  "<r_N>"
  Bus Selector3/2 -> Gain8/1  "<v_N>"
  Bus Creator3/1 -> Bus Creator1/3  "Cube3_estState"
  Bus Selector3/4 -> Gain11/1  "<w_BN>"
  Gain/1 -> Bus Creator/1
  Gain1/1 -> Bus Creator/2
  Gain2/1 -> Bus Creator/3
  Gain3/1 -> Bus Creator/4
  Gain4/1 -> Bus Creator2/1  "r_N_est"
  Gain5/1 -> Bus Creator2/2  "v_N_est"
  Gain6/1 -> Bus Creator2/3  "q_BN_est"
  Gain7/1 -> Bus Creator2/4  "w_BN_est"
  Gain8/1 -> Bus Creator3/2
  Gain9/1 -> Bus Creator3/1
  Gain10/1 -> Bus Creator3/3
  Gain11/1 -> Bus Creator3/4
  Constant/1 -> Quat IC Override/2
  Quat IC Override1/1 -> Display/1, Scope/2, [q2C]
  [q2] -> Quat IC Override1/1, Display1/1, Scope/1
  Constant1/1 -> Quat IC Override1/2
  Constant2/1 -> Quat IC Override2/2
  Bus Selector/3 -> [q1]  "<q1_BN>"
  [q1C] -> Gain2/1
  Bus Selector/4 -> Gain3/1  "<w_BN>"
  Bus Selector2/3 -> [q2]  "<q1_BN>"
  [q2C] -> Gain6/1
  Bus Selector3/3 -> [q3]  "<q1_BN>"
  [q3C] -> Gain10/1
  Quat IC Override2/1 -> Scope1/2, [q3C]
  [q3] -> Scope1/1, Quat IC Override2/1
  Quat IC Override/1 -> Scope2/2, [q1C]
  [q1] -> Scope2/1, Quat IC Override/1

== system Main1/NEW/Flight Computers1/Subsystem ==
  note: Torquer Shunts
  note: Sensor Ak Signals
  PwbMEXin : Inport
  Acc1 : Constant
  Acc2 : Constant
  Bus Creator{,3..5} (4 alike) : BusCreator  Inputs=2
  Bus Creator1 : BusCreator  Inputs=8
  Bus Creator2 : BusCreator  Inputs=3
  Chart : Subsystem  TreatAsAtomicUnit=on
  Clock : Clock
  Constant : Constant  Value=OpModes
  Constant1 : Constant  Value=OpTimes
  Constant2 : Constant  Value=SeperationTime
  Constant3 : Constant
  Constant4 : Constant
  Constant5 : Constant
  Gyro1 : Constant
  Gyro2 : Constant
  Mag1 : Constant
  Mag2 : Constant
  SunSensor1 : Constant
  SunSensor2 : Constant
  Ground Commands : Outport
  Pwbrd : Outport  Port=2
  wires:
  PwbMEXin/1 -> Chart/1(PwbMEX)
  Clock/1 -> Chart/2(time)  "time"
  Constant2/1 -> Chart/5(SeparationTime)  "SeparationTime"
  Constant1/1 -> Chart/3(OpTimes)  "OpTimes"
  Constant/1 -> Chart/4(OpModes)  "OpModes"
  Constant5/1 -> Bus Creator2/2  "TC_Y1"
  SunSensor1/1 -> Bus Creator1/7  "SunS1Ak"
  SunSensor2/1 -> Bus Creator1/8  "SunS2Ak"
  Gyro1/1 -> Bus Creator1/5  "Gyro1Ak"
  Bus Creator4/1 -> Pwbrd/1
  Gyro2/1 -> Bus Creator1/6  "Gyro2Ak"
  Mag2/1 -> Bus Creator1/2  "Mag2Ak"
  Constant3/1 -> Bus Creator2/1  "TC_X1"
  Bus Creator/1 -> Bus Creator4/1  "PwbrdCmmds"
  Bus Creator1/1 -> Bus Creator3/1  "SensorsAk"
  Bus Creator3/1 -> Bus Creator4/2  "ADCSAks"
  Chart/1(OM) -> Bus Creator5/1, Bus Creator/1  "OpMode"
  Acc1/1 -> Bus Creator1/3  "Accel1Ak"
  Chart/2(SEPC) -> Bus Creator5/2, Bus Creator/2  "SepCmd"
  Bus Creator2/1 -> Bus Creator3/2  "TorquerAk"
  Acc2/1 -> Bus Creator1/4  "Accel2Ak"
  Mag1/1 -> Bus Creator1/1  "Mag1Ak"
  Constant4/1 -> Bus Creator2/3  "TC_Z1"
  Bus Creator5/1 -> Ground Commands/1

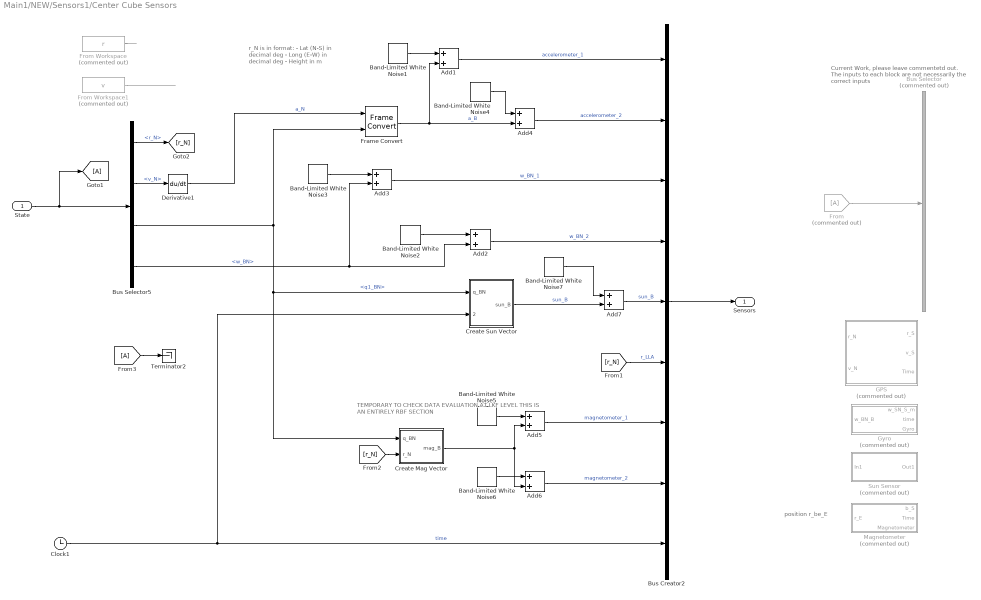
== system Main1/NEW/Sensors1/Center Cube Sensors ==
  note: position r_be_E
  note: Current Work, please leave commentetd out.
      | The inputs to each block are not necessarily
      | the correct inputs
  note: TEMPORARY TO CHECK DATA EVALUATION AT LKF LEVEL
      | THIS IS AN ENTIRELY RBF SECTION
  note: r_N is in format:
      | - Lat (N-S) in decimal deg
      | - Long (E-W) in decimal deg
      | - Height in m
  State : Inport
  Add{1..7} (7 alike) : Sum
  Band-Limited White Noise1 : simulink/Sources/Band-Limited White Noise  Cov=[0.1]  Ts=st  seed=[23341]
  Band-Limited White Noise{2..3,5..7} (5 alike) : simulink/Sources/Band-Limited White Noise  Cov=[0.1]  Ts=0.1  seed=[23341]
  Band-Limited White Noise4 : simulink/Sources/Band-Limited White Noise  Cov=[0.1]  Ts=st  seed=[23341]
  Bus Creator2 : BusCreator  Inputs=9
  Bus Selector : BusSelector  Commented=on  OutputSignals=r_N,v_N,q_BN,w_BN
  Bus Selector5 : BusSelector  OutputSignals=r_N,v_N,q1_BN,w_BN
  Clock1 : Clock
  Create Mag Vector : Subsystem
  Create Sun Vector : Subsystem  AncestorBlock=SimMainLibrary/SideCubeSensors/Create Sun Vector
  Derivative1 : Derivative  CoefficientInTFapproximation=.01
  Frame Convert : SimMainLibrary/SideCubeSensors/Frame Convert
      settings: SourceProductName=CUGravity Library
  From : From  Commented=on
  From Workspace : FromWorkspace  Commented=on  VariableName=r  SampleTime=0
  From Workspace1 : FromWorkspace  Commented=on  VariableName=v  SampleTime=0
  GPS : Subsystem  Commented=on
  Gyro : Subsystem  Commented=on
  Magnetometer : Subsystem  Commented=on
  Sun Sensor : Subsystem  Commented=on
  Terminator2 : Terminator
  Sensors : Outport
  wires:
  Bus Selector5/1 -> [r_N]  "<r_N>"
  Add1/1 -> Bus Creator2/1  "accelerometer_1"
  Bus Selector5/2 -> Derivative1/1  "<v_N>"
  Band-Limited White Noise1/1 -> Add1/1
  Frame Convert/1 -> Add4/2, Add1/2  "a_B"
  Add4/1 -> Bus Creator2/2  "accelerometer_2"
  Band-Limited White Noise2/1 -> Add2/1
  Band-Limited White Noise3/1 -> Add3/1
  Bus Selector5/4 -> Add3/2, Add2/2  "<w_BN>"
  State/1 -> [A], Bus Selector5/1
  Bus Creator2/1 -> Sensors/1
  Band-Limited White Noise4/1 -> Add4/1
  Add7/1 -> Bus Creator2/5  "sun_B"
  Clock1/1 -> Create Sun Vector/2(GPS time), Bus Creator2/9  "time"
  Add2/1 -> Bus Creator2/4  "w_BN_2"
  Add3/1 -> Bus Creator2/3  "w_BN_1"
  Band-Limited White Noise7/1 -> Add7/1
  Create Sun Vector/1(sun_B) -> Add7/2  "sun_B"
  [r_N] -> Bus Creator2/6  "r_LLA"
  Add6/1 -> Bus Creator2/8  "magnetometer_2"
  Create Mag Vector/1(mag_B) -> Add6/2, Add5/2
  Band-Limited White Noise6/1 -> Add6/1
  Add5/1 -> Bus Creator2/7  "magnetometer_1"
  Bus Selector5/3 -> Create Mag Vector/1(q_BN), Create Sun Vector/1(q_BN), Frame Convert/2  "<q1_BN>"
  Band-Limited White Noise5/1 -> Add5/1
  [r_N] -> Create Mag Vector/2(r_N)
  From/1 -> Bus Selector/1
  From Workspace1/1 -> ?
  From Workspace/1 -> ?
  Derivative1/1 -> Frame Convert/1  "a_N"
  [A] -> Terminator2/1

== system Main1/NEW/Sensors1/EndSat Sensor1 ==
  note: Things to Check:
      | Make sure that q1_BN is quaternion of B relative to N, otherwise rotation may be in the wrong direction.
      | Need to get an accurate measurement of B_N in order to calculate B_B.
      | Need to test the calculation to find the sun vector in the B frame.
  note: Add Noise
  State : Inport
  Acceleration N->B frame : aerolibutil/Quaternion Rotation
  Add{1..2,4,6} (4 alike) : Sum  Inputs=|++
  Add3 : Sum  Inputs=++|
  Add5 : Sum  Inputs=++|
  Add8 : Sum  Inputs=++|
  Band-Limited White Noise{1..7} (7 alike) : simulink/Sources/Band-Limited White Noise  Cov=[0.1]  Ts=0.1  seed=[23341]
  Bus Creator2 : BusCreator  Inputs=7
  Bus Selector5 : BusSelector  OutputSignals=r_N,v_N,q1_BN,w_BN
  Clock : Clock
  Create Sun Vector : SimMainLibrary/SideCubeSensors/Create Sun Vector
      settings: SourceProductName=CUGravity Library
  Magnetic Field Vector N frame : FromWorkspace  VariableName=B_N  SampleTime=0
  Magnetic Field Vector N->B frame : aerolibutil/Quaternion Rotation
  vel to acc : Derivative  CoefficientInTFapproximation=.01
  Sensors : Outport
  wires:
  Bus Selector5/1 -> Create Sun Vector/2  "<r_N>"
  Add8/1 -> Bus Creator2/2  "accelerometer_2"
  Band-Limited White Noise6/1 -> Add5/2
  Band-Limited White Noise5/1 -> Add4/1
  State/1 -> Bus Selector5/1
  Bus Selector5/2 -> vel to acc/1  "<v_N>"
  Band-Limited White Noise1/1 -> Add1/1
  Add1/1 -> Bus Creator2/1  "accelerometer_1"
  Add4/1 -> Bus Creator2/3  "magnetometer_1"
  Magnetic Field Vector N->B frame/1 -> Add5/1, Add4/2  "B_B"
  Bus Creator2/1 -> Sensors/1
  Bus Selector5/3 -> Create Sun Vector/1, Magnetic Field Vector N->B frame/1, Acceleration N->B frame/1  "<q1_BN>"
  Bus Selector5/4 -> Add3/1, Add2/2  "<w_BN>"
  Band-Limited White Noise4/1 -> Add8/2
  Add3/1 -> Bus Creator2/6  "w_BN_2"
  Add5/1 -> Bus Creator2/4  "magnetometer_2"
  Add2/1 -> Bus Creator2/5  "w_BN_1"
  Add6/1 -> Bus Creator2/7  "sun_B"
  Band-Limited White Noise7/1 -> Add6/2
  Create Sun Vector/1 -> Add6/1
  Band-Limited White Noise2/1 -> Add2/1
  Band-Limited White Noise3/1 -> Add3/2
  Acceleration N->B frame/1 -> Add1/2, Add8/1  "a_B"
  vel to acc/1 -> Acceleration N->B frame/2  "a_N"
  Magnetic Field Vector N frame/1 -> Magnetic Field Vector N->B frame/2
  Clock/1 -> Create Sun Vector/3

== system Main1/NEW/Sensors1/EndSat Sensor2 ==
  note: Things to Check:
      | Make sure that q1_BN is quaternion of B relative to N, otherwise rotation may be in the wrong direction.
      | Need to get an accurate measurement of B_N in order to calculate B_B.
      | Need to test the calculation to find the sun vector in the B frame.
  note: Add Sensor Noise
  State : Inport
  Acceleration N->B frame : aerolibutil/Quaternion Rotation
  Add{1..2,4,6} (4 alike) : Sum  Inputs=|++
  Add3 : Sum  Inputs=++|
  Add5 : Sum  Inputs=++|
  Add8 : Sum  Inputs=++|
  Band-Limited White Noise{1..7} (7 alike) : simulink/Sources/Band-Limited White Noise  Cov=[0.1]  Ts=0.1  seed=[23341]
  Bus Creator2 : BusCreator  Inputs=7
  Bus Selector5 : BusSelector  OutputSignals=v_N,q1_BN,w_BN,r_N
  Clock : Clock
  Create Sun Vector : SimMainLibrary/SideCubeSensors/Create Sun Vector
      settings: SourceProductName=CUGravity Library
  Magnetic Field Vector N frame : FromWorkspace  VariableName=B_N  SampleTime=0
  Magnetic Field Vector N->B frame : aerolibutil/Quaternion Rotation
  vel to acc : Derivative  CoefficientInTFapproximation=.01
  Sensors : Outport
  wires:
  Bus Selector5/4 -> Create Sun Vector/2  "<r_N>"
  Add8/1 -> Bus Creator2/2  "accelerometer_2"
  Band-Limited White Noise6/1 -> Add5/2
  Band-Limited White Noise5/1 -> Add4/1
  State/1 -> Bus Selector5/1
  Bus Selector5/1 -> vel to acc/1  "<v_N>"
  Band-Limited White Noise1/1 -> Add1/1
  Add1/1 -> Bus Creator2/1  "accelerometer_1"
  Add4/1 -> Bus Creator2/3  "magnetometer_1"
  Magnetic Field Vector N->B frame/1 -> Add5/1, Add4/2  "B_B"
  Bus Creator2/1 -> Sensors/1
  Bus Selector5/2 -> Create Sun Vector/1, Magnetic Field Vector N->B frame/1, Acceleration N->B frame/1  "<q1_BN>"
  Bus Selector5/3 -> Add2/2, Add3/1  "<w_BN>"
  Band-Limited White Noise4/1 -> Add8/2
  Add3/1 -> Bus Creator2/6  "w_BN_2"
  Add5/1 -> Bus Creator2/4  "magnetometer_2"
  Add2/1 -> Bus Creator2/5  "w_BN_1"
  Add6/1 -> Bus Creator2/7  "sun_B"
  Band-Limited White Noise7/1 -> Add6/2
  Create Sun Vector/1 -> Add6/1
  Band-Limited White Noise2/1 -> Add2/1
  Band-Limited White Noise3/1 -> Add3/2
  Acceleration N->B frame/1 -> Add1/2, Add8/1  "a_B"
  vel to acc/1 -> Acceleration N->B frame/2  "a_N"
  Magnetic Field Vector N frame/1 -> Magnetic Field Vector N->B frame/2
  Clock/1 -> Create Sun Vector/3

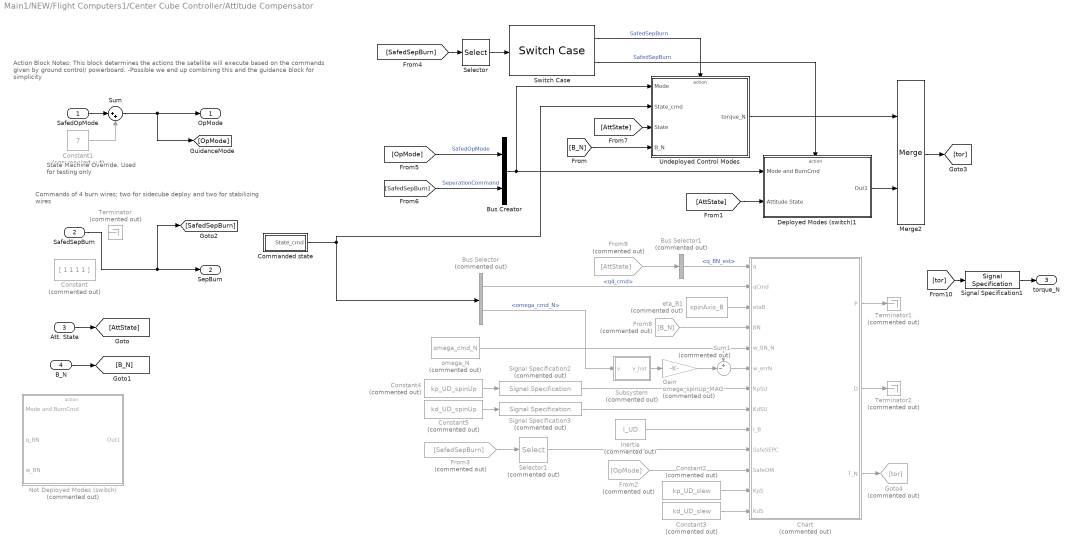
== system Main1/NEW/Flight Computers1/Center Cube Controller/Attitude Compensator ==
  note: State Machine Override. Used for testing only
  note: Commands of 4 burn wires; two for sidecube deploy
      | and two for stabilizing wires
  note: Action Block
      | Notes: This block determines the actions the satellite will execute based on the commands given by ground control/ powerboard.
      | -Possible we end up combining this and the guidance block for simplicity
  SafedOpMode : Inport
  SafedSepBurn : Inport  Port=2
  Att. State : Inport  Port=3
  B_N : Inport  Port=4
  Bus Creator : BusCreator  Inputs=2
  Bus Selector : BusSelector  Commented=on  OutputSignals=q4_cmd,omega_cmd_N
  Bus Selector1 : BusSelector  Commented=on  OutputSignals=q_BN_est
  Chart : Subsystem  Commented=on  TreatAsAtomicUnit=on
  Commanded state : Subsystem
  Constant : Constant  Commented=on  Value=[ 1 1 1 1 ]
  Constant1 : Constant  Commented=on  Value=7
  Constant2 : Constant  Commented=on  Value=kp_UD_slew
  Constant3 : Constant  Commented=on  Value=kd_UD_slew
  Constant4 : Constant  Commented=on  Value=kp_UD_spinUp
  Constant5 : Constant  Commented=on  Value=kd_UD_spinUp
  Deployed Modes (switch)1 : Subsystem
  From2 : From  Commented=on  GotoTag=OpMode
  From3 : From  Commented=on  GotoTag=SafedSepBurn
  From8 : From  Commented=on  GotoTag=B_N
  From9 : From  Commented=on  GotoTag=AttState
  Gain : Gain  Commented=on  Gain=omega_spinUp_MAG
  Goto4 : Goto  Commented=on  GotoTag=tor
  Inertia : Constant  Commented=on  Value=I_UD
  Merge2 : Merge
  Not Deployed Modes (switch) : Subsystem  Commented=on
  Selector : Selector  InputPortWidth=4  IndexOptions=Index vector (dialog)  Indices=[1]  OutputSizes=1
  Selector1 : Selector  Commented=on  InputPortWidth=4  IndexOptions=Index vector (dialog)  Indices=[1]  OutputSizes=1
  Signal Specification1 : SignalSpecification  OutDataTypeStr=double  Dimensions=3
  Signal Specification2 : SignalSpecification  Commented=on  OutDataTypeStr=double  Dimensions=1
  Signal Specification3 : SignalSpecification  Commented=on  OutDataTypeStr=double  Dimensions=1
  Subsystem : Subsystem  Commented=on
  Sum : Sum  Inputs=|++
  Sum1 : Sum  Commented=on  Inputs=+-|
  Switch Case : SwitchCase  CaseConditions={0,1}  ShowDefaultCase=off
  Terminator : Terminator  Commented=on
  Terminator1 : Terminator  Commented=on
  Terminator2 : Terminator  Commented=on
  Undeployed Control Modes : Subsystem
  eta_B1 : Constant  Commented=on  Value=spinAxis_B
  omega_N : Constant  Commented=on  Value=omega_cmd_N
  OpMode : Outport
  SepBurn : Outport  Port=2
  torque_N : Outport  Port=3
  wires:
  Sum/1 -> [OpMode], OpMode/1
  Undeployed Control Modes/1(torque_N) -> Merge2/1
  Deployed Modes (switch)1/1(Out1) -> Merge2/2
  [SafedSepBurn] -> Selector/1
  SafedSepBurn/1 -> SepBurn/1, [SafedSepBurn]
  Switch Case/1 -> Undeployed Control Modes/Action  "SafedSepBurn"
  Switch Case/2 -> Deployed Modes (switch)1/Action  "SafedSepBurn"
  [OpMode] -> Bus Creator/1  "SafedOpMode"
  Bus Creator/1 -> Undeployed Control Modes/1(Mode), Deployed Modes (switch)1/1(Mode and BurnCmd)
  [SafedSepBurn] -> Bus Creator/2  "SeperationCommand"
  [AttState] -> Undeployed Control Modes/3(State)
  [AttState] -> Deployed Modes (switch)1/2(Attitude State)
  Att. State/1 -> [AttState]
  B_N/1 -> [B_N]
  [B_N] -> Undeployed Control Modes/4(B_N)
  Signal Specification1/1 -> torque_N/1
  SafedOpMode/1 -> Sum/1
  Constant1/1 -> Sum/2
  Selector/1 -> Switch Case/1
  Gain/1 -> Sum1/2
  omega_N/1 -> Sum1/1, Chart/5(w_BN_N)
  Subsystem/1(v_hat) -> Gain/1
  Sum1/1 -> Chart/6(w_errN)
  Chart/1(P) -> Terminator1/1
  Chart/2(D) -> Terminator2/1
  Merge2/1 -> [tor]
  From2/1 -> Chart/11(SafeOM)
  From3/1 -> Selector1/1
  Inertia/1 -> Chart/9(I_B)
  Constant5/1 -> Signal Specification3/1
  Constant4/1 -> Signal Specification2/1
  Commanded state/1(State_cmd) -> Bus Selector/1, Undeployed Control Modes/2(State_cmd)
  Bus Selector/1 -> Chart/2(qCmd)  "<q4_cmd>"
  Bus Selector/2 -> Subsystem/1(v)  "<omega_cmd_N>"
  Constant2/1 -> Chart/12(KpS)
  Constant3/1 -> Chart/13(KdS)
  Signal Specification2/1 -> Chart/7(KpSU)
  Signal Specification3/1 -> Chart/8(KdSU)
  eta_B1/1 -> Chart/3(etaB)
  From8/1 -> Chart/4(BN)
  Bus Selector1/1 -> Chart/1(q)  "<q_BN_est>"
  From9/1 -> Bus Selector1/1
  Chart/3(T_N) -> Goto4/1
  [tor] -> Signal Specification1/1
  Selector1/1 -> Chart/10(SafeSEPC)

== system Main1/NEW/Flight Computers1/Center Cube Controller/Motor Control Placeholder ==
  note: Tether Control Sybsystem
      | When the spin rate of the CubeSat reaches
      | 6rpm, the tether will unreel a set amount
  spin rate : Inport
  SafedOpMode : Inport  Port=2
  If : If  NumInputs=2  IfExpression=u1 > 5 & u2 > 0
  Math Function : Math  Operator=square  SaturateOnIntegerOverflow=on
  Merge : Merge
  Mux : Mux  Commented=on  Inputs=2
  Spinning fast : Subsystem  TreatAsAtomicUnit=on
  Spinning slow : Subsystem  TreatAsAtomicUnit=on
  Sqrt : Sqrt  SaturateOnIntegerOverflow=on
  Sum of Elements : Sum  Inputs=+
  motor cmd : Outport
  wires:
  Math Function/1 -> Sum of Elements/1
  Sum of Elements/1 -> Sqrt/1
  spin rate/1 -> Math Function/1
  Sqrt/1 -> If/1
  Spinning fast/1(Out1) -> Merge/1
  Spinning slow/1(Out1) -> Merge/2
  If/1 -> Spinning fast/Action
  If/2 -> Spinning slow/Action
  SafedOpMode/1 -> If/2
  Mux/1 -> ?
  Merge/1 -> motor cmd/1, Mux/2, Mux/1

== system Main1/NEW/Flight Computers1/Center Cube Controller/SafeMode ==
  note: Safe Mode Filter
  GrndCmds : Inport
  EstState : Inport  Port=2
  Safe Mode In : Inport  Port=3
  Pwbrd : Inport  Port=4
  "EKFhs " : Inport  Port=5
  Bus Creator : BusCreator  Inputs=2
  Bus Selector : BusSelector  OutputSignals=OpMode,SepCmd
  Bus Selector1 : BusSelector  OutputSignals=r_N_est,v_N_est,q_BN_est,w_BN_est
  Bus Selector2 : BusSelector  OutputSignals=PwbrdCmmds.OpMode,ADCSAks.SensorsAk.Mag1Ak,ADCSAks.SensorsAk.Mag2Ak,ADCSAks.SensorsAk.Accel1Ak,ADCSAks.SensorsAk.Accel2Ak,ADCSAks.SensorsAk.Gyro1Ak,ADCSAks.SensorsAk.Gyro2Ak,ADCSAks.SensorsAk.SunS1Ak,ADCSAks.SensorsAk.SunS2Ak,ADCSAks.TorquerAk.TC_X1,ADCSAks.TorquerAk.TC_Y1,ADCSAks.TorquerAk.TC_Z1
  Bus Selector4 : BusSelector  OutputSignals=Cube2_estState
  Chart1 : Subsystem  TreatAsAtomicUnit=on  mask(Operation Logic){}
      mask help:
      | This system acts as a state machine (for ACS) which determines the switching logic between modes, based on component level errors or calculated Safe Mode. The chart performs two (2) main operations:
      |
      | First, it takes the Ak measurements for each sensor (magnetometer, gyro, accelerometer, sun sensor, and magnetorquers), and determines whether the sensors are working properly. The state machine is notified if any are not within normal safe operation requirements.
      |
      | Second (state machine), using this functionality as well as commands (power board and ground) and EKF estimation and status, the chart computes which mode of operation the satellite is in, the status of the operation (safe or not safe), and power board error messages. If the Safe Mode command output is false, then override operation is required.
  Clock : Clock
  Gain : Gain  Gain=[1;1;1;1]
  SafedOpMode : Outport
  SafedSeperationBurn : Outport  Port=2
  SafedPos : Outport  Port=3
  SafedVel : Outport  Port=4
  Safed Att. State : Outport  Port=5
  Safe Mode Out : Outport  Port=6
  PwbMEX : Outport  Port=7
  wires:
  Clock/1 -> Chart1/16(t)  "t"
  "EKFhs "/1 -> Chart1/14(EKFhs)  "EKFhs"
  Bus Selector1/4 -> Bus Creator/2  "<w_BN_est>"
  Bus Selector1/2 -> SafedVel/1  "<v_N_est>"
  Bus Selector1/1 -> SafedPos/1  "<r_N_est>"
  EstState/1 -> Bus Selector4/1
  GrndCmds/1 -> Bus Selector/1
  Safe Mode In/1 -> Chart1/15(SafeMode_In)  "SafeMode_In"
  Chart1/3(SafeMode_Out) -> Safe Mode Out/1
  Bus Selector/2 -> Gain/1, Chart1/18(SeperationCommand)  "<SepCmd>"
  Pwbrd/1 -> Bus Selector2/1
  Bus Selector2/1 -> Chart1/1(PbOpMode)  "<OpMode>"
  Chart1/1(OpMode_Out) -> SafedOpMode/1
  Chart1/2(PwbMEX) -> PwbMEX/1
  Bus Selector1/3 -> Bus Creator/1  "<q_BN_est>"
  Bus Selector4/1 -> Bus Selector1/1, Chart1/13(EKFAE)  "<Cube2_estState>"
  Bus Creator/1 -> Safed Att. State/1
  Bus Selector/1 -> Chart1/17(OpMode)  "<OpMode>"
  Gain/1 -> SafedSeperationBurn/1
  Bus Selector2/2 -> Chart1/2(Mag1)  "<Mag1Ak>"
  Bus Selector2/3 -> Chart1/3(Mag2)  "<Mag2Ak>"
  Bus Selector2/4 -> Chart1/4(Acc1)  "<Accel1Ak>"
  Bus Selector2/5 -> Chart1/5(Acc2)  "<Accel2Ak>"
  Bus Selector2/6 -> Chart1/6(Gyro1)  "<Gyro1Ak>"
  Bus Selector2/7 -> Chart1/7(Gyro2)  "<Gyro2Ak>"
  Bus Selector2/8 -> Chart1/8(Sun1)  "<SunS1Ak>"
  Bus Selector2/9 -> Chart1/9(Sun2)  "<SunS2Ak>"
  Bus Selector2/10 -> Chart1/10(MagX1)  "<TC_X1>"
  Bus Selector2/11 -> Chart1/11(MagY1)  "<TC_Y1>"
  Bus Selector2/12 -> Chart1/12(MagZ1)  "<TC_Z1>"

== system Main1/NEW/Flight Computers1/Center Cube Controller/Torque Coil Management ==
  note: Navigation Block
      | This block takes in data from the Actions/guidance block as to the current attitude of the spacecraft, the desired attitude of the spacecraft, and the required torque and outputs the current necessary to be applied to the torque coils as well as the torque currently being applied by the torque coils.
  Att. State : Inport
  torque_N : Inport  Port=2
  B_N : Inport  Port=3
  Bus Selector : BusSelector  OutputSignals=q_BN_est
  Quat1_to_Quat4 : SimMainLibrary/Quat1_to_Quat4
      settings: SourceProductName=CUGravity Library
  Torque Coil Management : Subsystem  TreatAsAtomicUnit=on
  CenterCube_PWM_cmds : Outport
  torque_coils : Outport  Port=2
  wires:
  torque_N/1 -> Torque Coil Management/1(torque_cmd_N)
  B_N/1 -> Torque Coil Management/3(B_N)
  Att. State/1 -> Bus Selector/1
  Bus Selector/1 -> Quat1_to_Quat4/1  "<q_BN_est>"
  Quat1_to_Quat4/1 -> Torque Coil Management/2(q4)
  Torque Coil Management/1(torque_N) -> torque_coils/1
  Torque Coil Management/2(I_coils) -> CenterCube_PWM_cmds/1
